simulink model "ElectromagneticSuspension_Simulink"  (R2021a)
settings: Solver=VariableStepAuto  StartTime=0.0  StopTime=10.0  RelTol=1e-3
values from neighbouring files (symbols this model uses):
  b1 = 500    [ElectromagneticSuspension_CodeMatlab.m]
  b2 = 1050    [ElectromagneticSuspension_CodeMatlab.m]
  k1 = 16812    [ElectromagneticSuspension_CodeMatlab.m]
  k2 = 190000    [ElectromagneticSuspension_CodeMatlab.m]
  m1 = 250    [ElectromagneticSuspension_CodeMatlab.m]
  m2 = 50    [ElectromagneticSuspension_CodeMatlab.m]
undefined symbols (not defined in the file or in its folder): LF
libraries: instrumentseriallib x3, etargetslib x1
settings Model: Creator=ASUS  LastModifiedBy=ASUS
settings SolverCC: AlgebraicLoopSolver=TrustRegion
settings SFSimCC: CustomCodeUndefinedFunction=UseInterfaceOnly

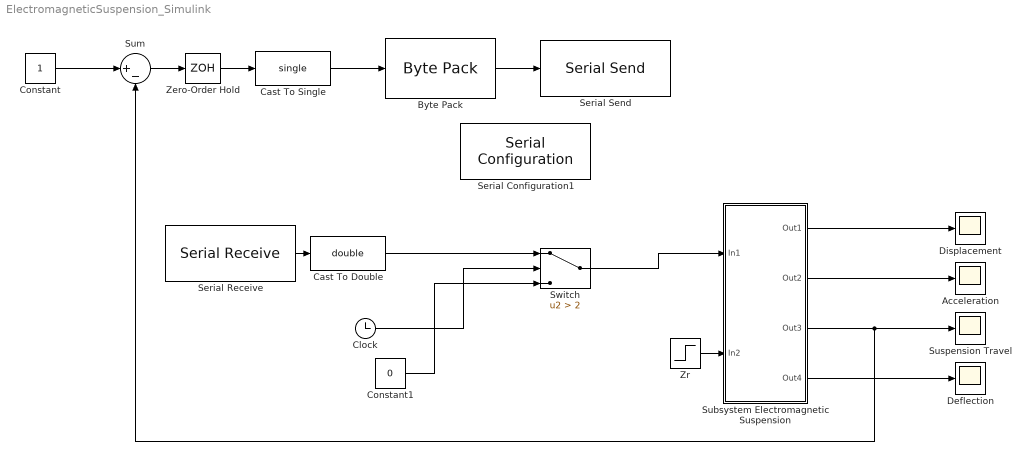
== system ElectromagneticSuspension_Simulink ==
  Acceleration : Scope
  Byte Pack : etargetslib/Byte Pack  datatypes={'single'}  byteAlign=1
  Cast To Double : DataTypeConversion  OutDataTypeStr=double
  Cast To Single : DataTypeConversion  OutDataTypeStr=single
  Clock : Clock
      settings: Decimation=5
  Constant : Constant
  Constant1 : Constant  Value=0
  Deflection : Scope
  Displacement : Scope
  Serial Configuration1 : instrumentseriallib/Serial Configuration  Priority=-200000  Port=<Select a port...>  ComPort=<Select a port...>  BaudRate=115200  DataBits=8  Parity=none  StopBits=1  ByteOrder=little-endian  FlowControl=none  Timeout=10  SimulateUsing=Interpreted execution  BlockInModel=on
  Serial Receive : instrumentseriallib/Serial Receive  Port=<Select a port...>  ComPort=<Select a port...>  DataType=single  SaveDataType=uint8  ToggleHeader=off  Header=[]  ToggleTerminator=on  Terminator=LF ('\n')  CustomTerminator=[]  ToggleDataSize=on  DataSize=[1 1]  EnableBlockingMode=on  ActionDataUnavailable=Output last received value  ActionWhenDataUnavailable=Output last received value  CustomValue=0  SampleTime=0.05  SimulateUsing=Interpreted execution  BlockInModel=on
  Serial Send : instrumentseriallib/Serial Send  Port=<Select a port...>  ComPort=<Select a port...>  Header=[]  Terminator=<none>  CustomTerminator=[]  EnableBlockingMode=on  SimulateUsing=Interpreted execution  BlockInModel=on
  Subsystem Electromagnetic Suspension : Subsystem
  Sum : Sum  Inputs=|+-
  Suspension Travel : Scope
  Switch : Switch  Criteria=u2 > Threshold  Threshold=2
  Zero-Order Hold : ZeroOrderHold  SampleTime=0.05
  Zr : Step  Time=0.1  SampleTime=0
  wires:
  Zr/1 -> Subsystem Electromagnetic Suspension/2(In2)
  Subsystem Electromagnetic Suspension/1(Out1) -> Displacement/1
  Subsystem Electromagnetic Suspension/2(Out2) -> Acceleration/1
  Subsystem Electromagnetic Suspension/3(Out3) -> Suspension Travel/1, Sum/2
  Subsystem Electromagnetic Suspension/4(Out4) -> Deflection/1
  Constant/1 -> Sum/1
  Sum/1 -> Zero-Order Hold/1
  Zero-Order Hold/1 -> Cast To Single/1
  Cast To Single/1 -> Byte Pack/1
  Byte Pack/1 -> Serial Send/1
  Serial Receive/1 -> Cast To Double/1
  Cast To Double/1 -> Switch/1
  Clock/1 -> Switch/2
  Constant1/1 -> Switch/3
  Switch/1 -> Subsystem Electromagnetic Suspension/1(In1)

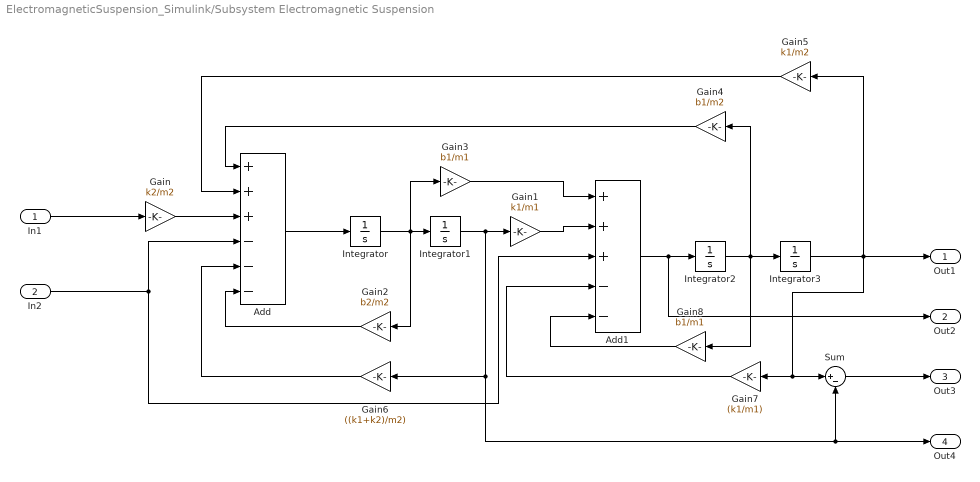
== system ElectromagneticSuspension_Simulink/Subsystem Electromagnetic Suspension ==
  In1 : Inport
  In2 : Inport  Port=2
  Add : Sum  Inputs=+++---
  Add1 : Sum  Inputs=+++--
  Gain : Gain  Gain=k2/m2
  Gain1 : Gain  Gain=k1/m1
  Gain2 : Gain  Gain=b2/m2
  Gain3 : Gain  Gain=b1/m1
  Gain4 : Gain  Gain=b1/m2
  Gain5 : Gain  Gain=k1/m2
  Gain6 : Gain  Gain=((k1+k2)/m2)
  Gain7 : Gain  Gain=(k1/m1)
  Gain8 : Gain  Gain=b1/m1
  Integrator : Integrator  LimitOutput=on  UpperSaturationLimit=10  LowerSaturationLimit=0
  Integrator1 : Integrator
  Integrator2 : Integrator
  Integrator3 : Integrator
  Sum : Sum  Inputs=|+-
  Out1 : Outport
  Out2 : Outport  Port=2
  Out3 : Outport  Port=3
  Out4 : Outport  Port=4
  wires:
  Gain8/1 -> Add1/5
  Gain2/1 -> Add/6
  Add1/1 -> Out2/1, Integrator2/1
  Gain4/1 -> Add/1
  Gain7/1 -> Add1/4
  Gain3/1 -> Add1/1
  Add/1 -> Integrator/1
  Integrator/1 -> Gain3/1, Gain2/1, Integrator1/1
  Integrator3/1 -> Out1/1, Gain5/1, Gain7/1, Sum/1
  Gain5/1 -> Add/2
  Integrator2/1 -> Gain8/1, Gain4/1, Integrator3/1
  Integrator1/1 -> Gain6/1, Out4/1, Sum/2, Gain1/1
  Gain1/1 -> Add1/2
  In2/1 -> Add1/3, Add/4
  Gain/1 -> Add/3
  Gain6/1 -> Add/5
  In1/1 -> Gain/1
  Sum/1 -> Out3/1
